simulink model "gm_IPCore_3Level_PWM"  (R2024a)
settings: Solver=VariableStepAuto  StartTime=0.0  StopTime=0.001  RelTol=1e-3
undefined symbols (not defined in the file or in its folder): f_Carrier, f_FPGA_clk, T_Carrier, T_FPGA_clk
libraries: hdlsllib x2
settings Model: PacingRate=0.100000  Creator=info  LastModifiedBy=info
settings OptimizationCC: BlockReduction=off  ConditionallyExecuteInputs=off  DefaultParameterBehavior=Inlined
settings DebuggingCC: AlgebraicLoopMsg=error  InheritedTsInSrcMsg=none  SingleTaskRateTransMsg=error
settings HardwareCC: ProdBitPerPointer=32  ProdBitPerSizeT=32  ProdBitPerPtrDiffT=32  ProdLargestAtomicFloat=None  ProdIntDivRoundTo=Undefined  ProdEndianess=Unspecified  ProdWordSize=32  ProdHWDeviceType=ASIC/FPGA->ASIC/FPGA  TargetBitPerPointer=64  TargetBitPerSizeT=64  TargetBitPerPtrDiffT=64  TargetLongLongMode=on  TargetIntDivRoundTo=Zero  TargetEndianess=LittleEndian  TargetWordSize=64  TargetHWDeviceType=Custom Processor->MATLAB Host Computer  ProdEqTarget=off

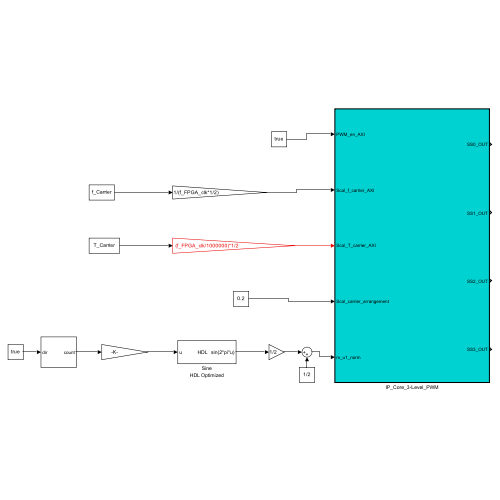
[thumbnail: Simulink's stored preview of the top-level diagram]
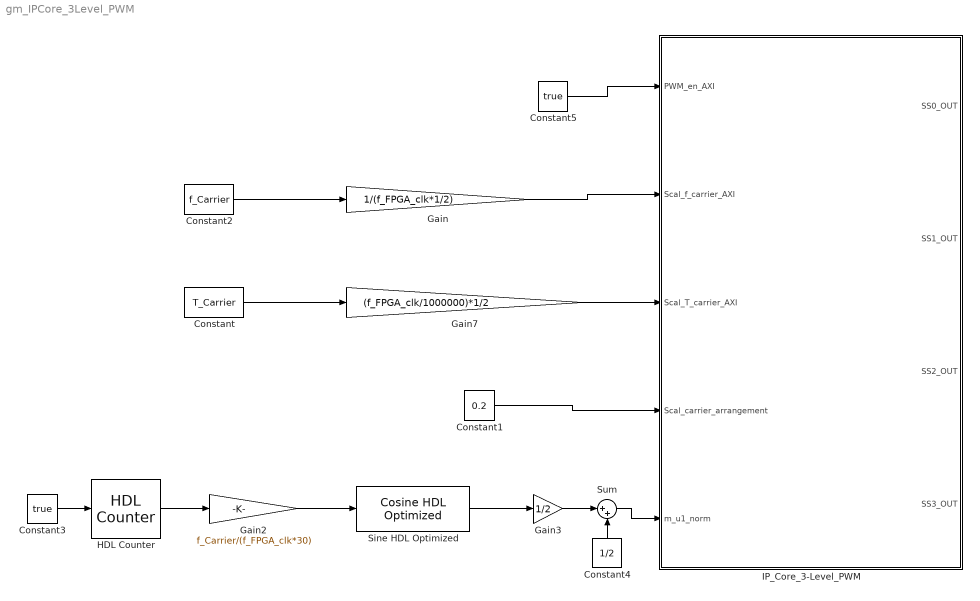
== system gm_IPCore_3Level_PWM ==
  Constant : Constant  Value=T_Carrier  SampleTime=T_FPGA_clk
  Constant1 : Constant  Value=0.2  OutDataTypeStr=double  SampleTime=T_FPGA_clk
  Constant2 : Constant  Value=f_Carrier  SampleTime=T_FPGA_clk
  Constant3 : Constant  Value=true  OutDataTypeStr=boolean  SampleTime=T_FPGA_clk
  Constant4 : Constant  Value=1/2  SampleTime=-1
  Constant5 : Constant  Value=true  SampleTime=-1
  Gain : Gain  Gain=1/(f_FPGA_clk*1/2)  OutDataTypeStr=fixdt(0,25,26)
  Gain2 : Gain  Gain=f_Carrier/(f_FPGA_clk*30)
  Gain3 : Gain  Gain=1/2
  Gain7 : Gain  Gain=(f_FPGA_clk/1000000)*1/2  OutDataTypeStr=fixdt(0,25,0)
  HDL Counter : hdlsllib/Sources/HDL Counter  CountType=Free running  CountInit=0  CountStep=1  CountMax=25  CountFromType=Initial value  CountFrom=0  CountResetPort=off  CountLoadPort=off  CountEnbPort=off  CountDirPort=on  CountHitOutputPort=off  CountDataType=Unsigned  CountWordLen=20  CountFracLen=0  CountSampTime=1
  IP_Core_3-Level_PWM : Subsystem  TreatAsAtomicUnit=on
  Sine HDL Optimized : hdlsllib/Lookup Tables/Cosine HDL Optimized  OutputFormula=sin(2*pi*u)  NumDataPoints=64  TableDataTypeStr=fixdt(0,16,15)  SimulateLUTROMDelay=off
      settings: LibrarySourceBlock=|
      | hdlsllib/Lookup
      | Tables/Sine
      | HDL Optimized
  Sum : Sum  Inputs=|++
  wires:
  Constant5/1 -> IP_Core_3-Level_PWM/1(PWM_en_AXI)
  Sum/1 -> IP_Core_3-Level_PWM/5(m_u1_norm)
  Gain3/1 -> Sum/1
  Constant4/1 -> Sum/2
  Constant3/1 -> HDL Counter/1
  HDL Counter/1 -> Gain2/1
  Gain2/1 -> Sine HDL Optimized/1
  Sine HDL Optimized/1 -> Gain3/1
  Constant1/1 -> IP_Core_3-Level_PWM/4(Scal_carrier_arrangement)
  Gain7/1 -> IP_Core_3-Level_PWM/3(Scal_T_carrier_AXI)
  Constant2/1 -> Gain/1
  Constant/1 -> Gain7/1
  Gain/1 -> IP_Core_3-Level_PWM/2(Scal_f_carrier_AXI)

== system gm_IPCore_3Level_PWM/IP_Core_3-Level_PWM ==
  note: Set pulse width in percent
  PWM_en_AXI : Inport  OutDataTypeStr=boolean  PortDimensions=1  SampleTime=1e-08
  Scal_f_carrier_AXI : Inport  Port=2  OutDataTypeStr=fixdt(0, 25, 26)  PortDimensions=1  SampleTime=1e-08
  Scal_T_carrier_AXI : Inport  Port=3  OutDataTypeStr=fixdt(0, 25, 0)  PortDimensions=1  SampleTime=1e-08
  Scal_carrier_arrangement : Inport  Port=4  OutDataTypeStr=double  PortDimensions=1  SampleTime=1e-08
  m_u1_norm : Inport  Port=5  OutDataTypeStr=double  PortDimensions=1  SampleTime=1e-08
  GenPWM : Subsystem
  Scal_f_carrier_AXI_term1 : Terminator
  SS0_OUT : Outport  SampleTime=1e-08  VectorParamsAs1DForOutWhenUnconnected=off
  SS1_OUT : Outport  Port=2  SampleTime=1e-08  VectorParamsAs1DForOutWhenUnconnected=off
  SS2_OUT : Outport  Port=3  SampleTime=1e-08  VectorParamsAs1DForOutWhenUnconnected=off
  SS3_OUT : Outport  Port=4  SampleTime=1e-08  VectorParamsAs1DForOutWhenUnconnected=off
  wires:
  PWM_en_AXI/1 -> GenPWM/1(PWM_en_AXI)
  Scal_f_carrier_AXI/1 -> Scal_f_carrier_AXI_term1/1
  Scal_T_carrier_AXI/1 -> GenPWM/2(Scal_T_carrier)
  Scal_carrier_arrangement/1 -> GenPWM/3(Scal_Carrier_arrangement)
  m_u1_norm/1 -> GenPWM/4(U1_norm)
  GenPWM/1(U1_S0) -> SS0_OUT/1
  GenPWM/2(U1_S1) -> SS1_OUT/1
  GenPWM/3(U1_S2) -> SS2_OUT/1
  GenPWM/4(U1_S3) -> SS3_OUT/1

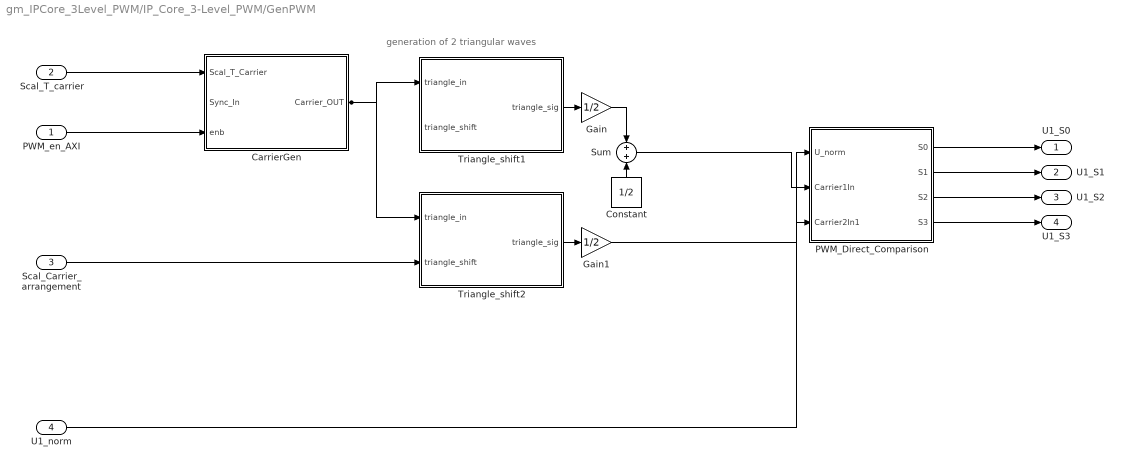
== system gm_IPCore_3Level_PWM/IP_Core_3-Level_PWM/GenPWM ==
  note: generation of 2 triangular waves
  PWM_en_AXI : Inport  OutDataTypeStr=boolean  PortDimensions=1  SampleTime=1e-08
  Scal_T_carrier : Inport  Port=2  OutDataTypeStr=fixdt(0, 25, 0)  PortDimensions=1  SampleTime=1e-08
  Scal_Carrier_arrangement : Inport  Port=3  OutDataTypeStr=double  PortDimensions=1  SampleTime=1e-08
  U1_norm : Inport  Port=4  OutDataTypeStr=double  PortDimensions=1  SampleTime=1e-08
  CarrierGen : Subsystem
  Constant : Constant  Value=1/2  OutDataTypeStr=fixdt(1,18,16)  SampleTime=T_FPGA_clk
  Gain : Gain  Gain=1/2  OutDataTypeStr=fixdt(1, 36, 33)
  Gain1 : Gain  Gain=1/2  OutDataTypeStr=fixdt(1, 36, 33)
  PWM_Direct_Comparison : Subsystem
  Sum : Sum  Inputs=+|+  OutDataTypeStr=fixdt(1, 37, 33)
  Triangle_shift1 : Subsystem
  Triangle_shift2 : Subsystem
  U1_S0 : Outport  SampleTime=1e-08
  U1_S1 : Outport  Port=2  SampleTime=1e-08
  U1_S2 : Outport  Port=3  SampleTime=1e-08
  U1_S3 : Outport  Port=4  SampleTime=1e-08
  wires:
  PWM_en_AXI/1 -> CarrierGen/3(enb)
  Scal_T_carrier/1 -> CarrierGen/1(Scal_T_Carrier)
  Scal_Carrier_arrangement/1 -> Triangle_shift2/2(triangle_shift)
  U1_norm/1 -> PWM_Direct_Comparison/1(U_norm)
  CarrierGen/1(Carrier_OUT) -> Triangle_shift1/1(triangle_in), Triangle_shift2/1(triangle_in)
  Constant/1 -> Sum/2
  Gain/1 -> Sum/1
  Gain1/1 -> PWM_Direct_Comparison/3(Carrier2In1)
  PWM_Direct_Comparison/1(S0) -> U1_S0/1
  PWM_Direct_Comparison/2(S1) -> U1_S1/1
  PWM_Direct_Comparison/3(S2) -> U1_S2/1
  PWM_Direct_Comparison/4(S3) -> U1_S3/1
  Sum/1 -> PWM_Direct_Comparison/2(Carrier1In)
  Triangle_shift1/1(triangle_sig) -> Gain/1
  Triangle_shift2/1(triangle_sig) -> Gain1/1

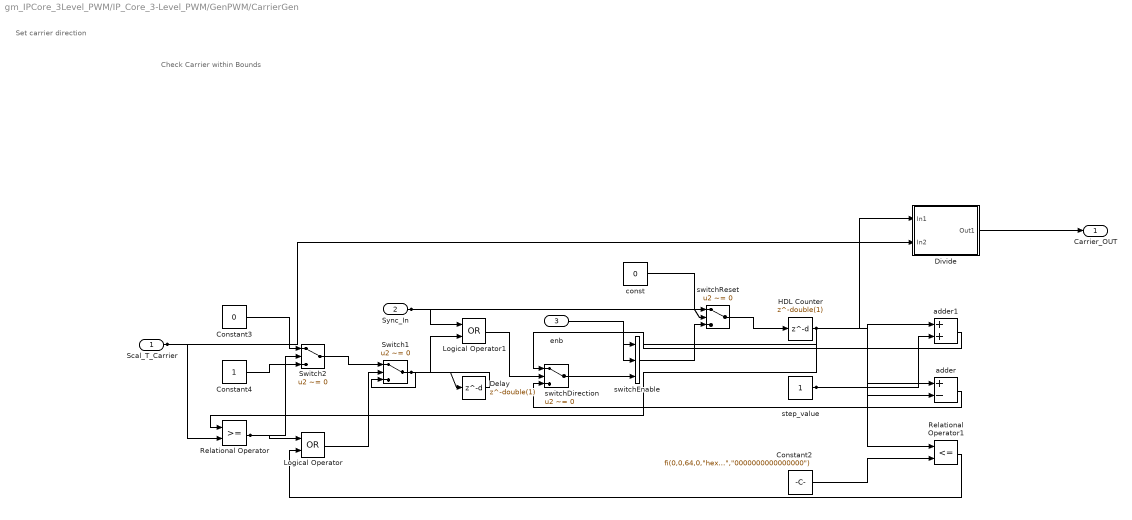
== system gm_IPCore_3Level_PWM/IP_Core_3-Level_PWM/GenPWM/CarrierGen ==
  note: Check Carrier within Bounds
  note: Set carrier direction
  Scal_T_Carrier : Inport  OutDataTypeStr=fixdt(0, 25, 0)  PortDimensions=1  SampleTime=1e-08
  Sync_In : Inport  Port=2  OutDataTypeStr=boolean  PortDimensions=1  SampleTime=1e-08
  enb : Inport  Port=3  OutDataTypeStr=boolean  PortDimensions=1  SampleTime=1e-08
  Constant2 : Constant  Value="fi(0,0,64,0,\"hex\",\"0000000000000000\")"  OutDataTypeStr=fixdt(0, 64, 0)  SampleTime=1e-08
  Constant3 : Constant  Value=0  OutDataTypeStr=boolean  SampleTime=1e-08
  Constant4 : Constant  OutDataTypeStr=boolean  SampleTime=1e-08
  Delay : Delay  DelayLength=double(1)  InitialCondition=0  SampleTime=1e-08
  Divide : Subsystem
  HDL Counter : Delay  DelayLength=double(1)  InitialCondition=0  SampleTime=1e-08
  Logical Operator : Logic  Operator=OR  AllPortsSameDT=off  OutDataTypeStr=boolean  SampleTime=1e-08
  Logical Operator1 : Logic  Operator=OR  AllPortsSameDT=off  OutDataTypeStr=boolean  SampleTime=1e-08
  Relational Operator : RelationalOperator  OutDataTypeStr=boolean  SampleTime=1e-08  InputSameDT=off
  Relational Operator1 : RelationalOperator  Operator=<=  OutDataTypeStr=boolean  SampleTime=1e-08  InputSameDT=off
  Switch1 : Switch  Criteria=u2 ~= 0  Threshold=double(0)  OutDataTypeStr=boolean  SampleTime=1e-08  SaturateOnIntegerOverflow=off  InputSameDT=off
  Switch2 : Switch  Criteria=u2 ~= 0  Threshold=double(0)  OutDataTypeStr=boolean  SampleTime=1e-08  SaturateOnIntegerOverflow=off  InputSameDT=off
  adder : Sum  Inputs=+-  OutDataTypeStr=fixdt(0, 20, 0)  AccumDataTypeStr=fixdt(0, 20, 0)  SampleTime=1e-08
  adder1 : Sum  OutDataTypeStr=fixdt(0, 20, 0)  AccumDataTypeStr=fixdt(0, 20, 0)  SampleTime=1e-08
  const : Constant  Value=0  VectorParams1D=off  OutDataTypeStr=fixdt(0, 20, 0)  SampleTime=1e-08
  step_value : Constant  VectorParams1D=off  OutDataTypeStr=fixdt(0, 20, 0)  SampleTime=1e-08
  switchDirection : Switch  Criteria=u2 ~= 0  Threshold=double(0)  OutDataTypeStr=fixdt(0, 20, 0)  SampleTime=1e-08  SaturateOnIntegerOverflow=off  InputSameDT=off
  switchEnable : MultiPortSwitch  DataPortOrder=Zero-based contiguous  Inputs=2  DiagnosticForDefault=None  zeroidx=on  OutDataTypeStr=fixdt(0, 20, 0)  SampleTime=1e-08  SaturateOnIntegerOverflow=off  InputSameDT=off
  switchReset : Switch  Criteria=u2 ~= 0  Threshold=double(0)  OutDataTypeStr=fixdt(0, 20, 0)  SampleTime=1e-08  SaturateOnIntegerOverflow=off  InputSameDT=off
  Carrier_OUT : Outport  SampleTime=1e-08
  wires:
  Scal_T_Carrier/1 -> Relational Operator/2, Divide/2(In2)
  Divide/1(Out1) -> Carrier_OUT/1
  HDL Counter/1 -> Relational Operator/1, Relational Operator1/1, adder1/1, adder/1, switchEnable/2, Divide/1(In1)
  Delay/1 -> Switch1/3
  step_value/1 -> adder1/2, adder/2
  Constant2/1 -> Relational Operator1/2
  Constant3/1 -> Switch2/1
  Constant4/1 -> Switch2/3
  Sync_In/1 -> switchReset/2, Logical Operator1/1
  enb/1 -> switchEnable/1
  const/1 -> switchReset/1
  Switch1/1 -> Delay/1, Logical Operator1/2
  switchReset/1 -> HDL Counter/1
  adder/1 -> switchDirection/3
  Relational Operator1/1 -> Logical Operator/2
  Logical Operator/1 -> Switch1/2
  Relational Operator/1 -> Switch2/2, Logical Operator/1
  Switch2/1 -> Switch1/1
  Logical Operator1/1 -> switchDirection/2
  adder1/1 -> switchDirection/1
  switchDirection/1 -> switchEnable/3
  switchEnable/1 -> switchReset/3

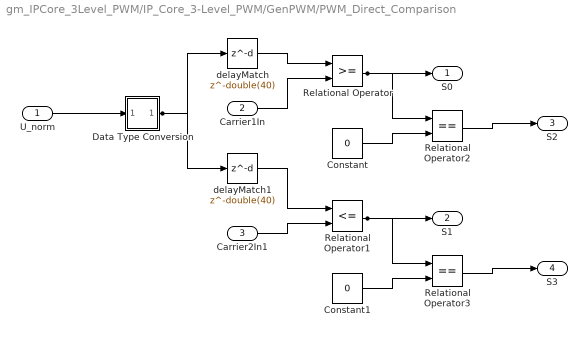
== system gm_IPCore_3Level_PWM/IP_Core_3-Level_PWM/GenPWM/PWM_Direct_Comparison ==
  U_norm : Inport  OutDataTypeStr=double  PortDimensions=1  SampleTime=1e-08
  Carrier1In : Inport  Port=2  OutDataTypeStr=fixdt(1, 37, 33)  PortDimensions=1  SampleTime=1e-08
  Carrier2In1 : Inport  Port=3  OutDataTypeStr=fixdt(1, 36, 33)  PortDimensions=1  SampleTime=1e-08
  Constant : Constant  Value=0  OutDataTypeStr=boolean  SampleTime=1e-08
  Constant1 : Constant  Value=0  OutDataTypeStr=boolean  SampleTime=1e-08
  Data Type Conversion : Subsystem
      mask Display: disp('NFP\nconv');
  Relational Operator : RelationalOperator  OutDataTypeStr=boolean  SampleTime=1e-08  InputSameDT=off
  Relational Operator1 : RelationalOperator  Operator=<=  OutDataTypeStr=boolean  SampleTime=1e-08  InputSameDT=off
  Relational Operator2 : RelationalOperator  Operator===  OutDataTypeStr=boolean  SampleTime=1e-08  InputSameDT=off
  Relational Operator3 : RelationalOperator  Operator===  OutDataTypeStr=boolean  SampleTime=1e-08  InputSameDT=off
  delayMatch : Delay  DelayLength=double(40)  InitialCondition=0  SampleTime=1e-08
  delayMatch1 : Delay  DelayLength=double(40)  InitialCondition=0  SampleTime=1e-08
  S0 : Outport  SampleTime=1e-08
  S1 : Outport  Port=2  SampleTime=1e-08
  S2 : Outport  Port=3  SampleTime=1e-08
  S3 : Outport  Port=4  SampleTime=1e-08
  wires:
  U_norm/1 -> Data Type Conversion/1(In1)
  Carrier1In/1 -> Relational Operator/2
  Carrier2In1/1 -> Relational Operator1/2
  Constant/1 -> Relational Operator2/2
  Constant1/1 -> Relational Operator3/2
  delayMatch/1 -> Relational Operator/1
  Relational Operator/1 -> Relational Operator2/1, S0/1
  Relational Operator1/1 -> Relational Operator3/1, S1/1
  Relational Operator2/1 -> S2/1
  Relational Operator3/1 -> S3/1
  Data Type Conversion/1(Out1) -> delayMatch1/1, delayMatch/1
  delayMatch1/1 -> Relational Operator1/1

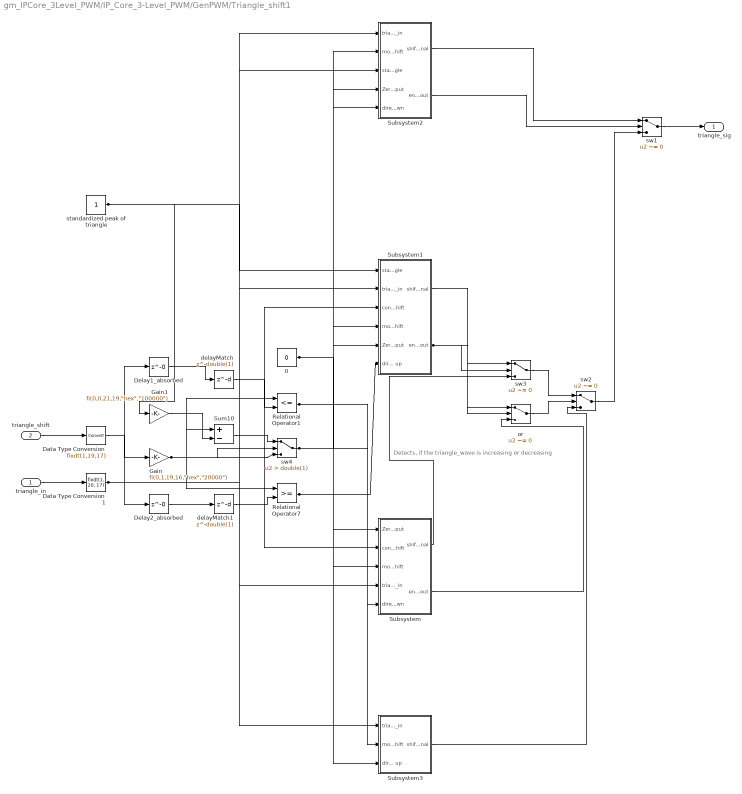
== system gm_IPCore_3Level_PWM/IP_Core_3-Level_PWM/GenPWM/Triangle_shift1 ==
  note: Detects, if the triangle_wave is increasing or decreasing
  triangle_in : Inport  OutDataTypeStr=fixdt(1, 18, 16)  PortDimensions=1  SampleTime=1e-08
  triangle_shift : Inport  Port=2  OutDataTypeStr=fixdt(1, 19, 17)  PortDimensions=1  SampleTime=1e-08
  0 : Constant  Value=0  OutDataTypeStr=boolean  SampleTime=1e-08
  Data Type Conversion : DataTypeConversion  OutDataTypeStr=fixdt(1,19,17)
  Data Type Conversion1 : DataTypeConversion  OutDataTypeStr=fixdt(1, 20, 17)  SampleTime=1e-08  SaturateOnIntegerOverflow=off  RndMeth=Floor
  Delay1_absorbed : Delay  DelayLength=0
  Delay2_absorbed : Delay  DelayLength=0
  Gain : Gain  Gain="fi(0,1,19,16,\"hex\",\"20000\")"  ParamDataTypeStr=fixdt(1, 19, 16)  OutDataTypeStr=fixdt(1, 20, 17)  SampleTime=1e-08
  Gain1 : Gain  Gain="fi(0,0,21,19,\"hex\",\"100000\")"  ParamDataTypeStr=fixdt(0, 21, 19)  OutDataTypeStr=fixdt(1, 20, 17)  SampleTime=1e-08
  Relational Operator1 : RelationalOperator  Operator=<=  OutDataTypeStr=boolean  SampleTime=1e-08  InputSameDT=off
  Relational Operator7 : RelationalOperator  OutDataTypeStr=boolean  SampleTime=1e-08  InputSameDT=off
  Subsystem : Subsystem
  Subsystem1 : Subsystem
  Subsystem2 : Subsystem
  Subsystem3 : Subsystem
  Sum10 : Sum  Inputs=+-  OutDataTypeStr=fixdt(1, 20, 17)  AccumDataTypeStr=fixdt(1, 21, 17)  SampleTime=1e-08
  delayMatch : Delay  DelayLength=double(1)  InitialCondition=0  SampleTime=1e-08
  delayMatch1 : Delay  DelayLength=double(1)  InitialCondition=0  SampleTime=1e-08
  or : Switch  Criteria=u2 ~= 0  Threshold=double(0)  OutDataTypeStr=boolean  SampleTime=1e-08  SaturateOnIntegerOverflow=off  InputSameDT=off
  standardized peak of triangle : Constant  OutDataTypeStr=fixdt(0, 21, 17)  SampleTime=1e-08
  sw1 : Switch  Criteria=u2 ~= 0  Threshold=double(0)  OutDataTypeStr=fixdt(1, 18, 16)  SampleTime=1e-08  SaturateOnIntegerOverflow=off  InputSameDT=off
  sw2 : Switch  Criteria=u2 ~= 0  Threshold=double(0)  OutDataTypeStr=fixdt(1, 21, 17)  SampleTime=1e-08  SaturateOnIntegerOverflow=off  InputSameDT=off
  sw3 : Switch  Criteria=u2 ~= 0  Threshold=double(0)  OutDataTypeStr=fixdt(1, 21, 17)  SampleTime=1e-08  SaturateOnIntegerOverflow=off  InputSameDT=off
  sw4 : Switch  Criteria=u2 > Threshold  Threshold=double(1)  OutDataTypeStr=fixdt(1, 20, 17)  SampleTime=1e-08  SaturateOnIntegerOverflow=off  InputSameDT=off
  triangle_sig : Outport  SampleTime=1e-08  VectorParamsAs1DForOutWhenUnconnected=off
  wires:
  triangle_in/1 -> Data Type Conversion1/1
  triangle_shift/1 -> Data Type Conversion/1
  0/1 -> Subsystem2/4(Zero_input), Subsystem1/5(Zero_input), Subsystem/1(Zero_input)
  Data Type Conversion/1 -> Gain/1
  Data Type Conversion1/1 -> Relational Operator7/1, Relational Operator1/1, Subsystem3/1(triangle_in), Subsystem2/1(triangle_in), Subsystem/4(triangle_in), Subsystem1/2(triangle_in), Delay1_absorbed/1, Delay2_absorbed/1
  delayMatch/1 -> Relational Operator1/2
  delayMatch1/1 -> Relational Operator7/2
  Gain/1 -> sw4/3, sw4/2, Sum10/1, Subsystem/2(converted triangle_shift), Subsystem1/3(converted triangle_shift)
  Gain1/1 -> Sum10/2
  Relational Operator1/1 -> Subsystem/5(direction down), Subsystem2/5(direction down)
  Relational Operator7/1 -> Subsystem1/6(direction up), Subsystem3/3(direction up)
  Subsystem/1(shifted triangle_in signal) -> sw3/3
  Subsystem/2(enable_out) -> or/3
  Subsystem1/1(shifted triangle_in signal) -> sw3/1
  Subsystem1/2(enable_out) -> sw3/2, or/2, or/1
  Subsystem2/1(shifted triangle_in signal) -> sw1/1
  Subsystem2/2(enable_out) -> sw1/2
  Subsystem3/1(shifted triangle_in signal) -> sw2/3
  Sum10/1 -> sw4/1
  or/1 -> sw2/2
  standardized peak of triangle/1 -> Gain1/1, Subsystem2/3(standardized peak of triangle), Subsystem1/1(standardized peak of triangle)
  sw1/1 -> triangle_sig/1
  sw2/1 -> sw1/3
  sw3/1 -> sw2/1
  sw4/1 -> Subsystem3/2(modified triangle_shift), Subsystem/3(modified triangle_shift), Subsystem1/4(modified triangle_shift), Subsystem2/2(modified triangle_shift)
  Delay1_absorbed/1 -> delayMatch/1
  Delay2_absorbed/1 -> delayMatch1/1

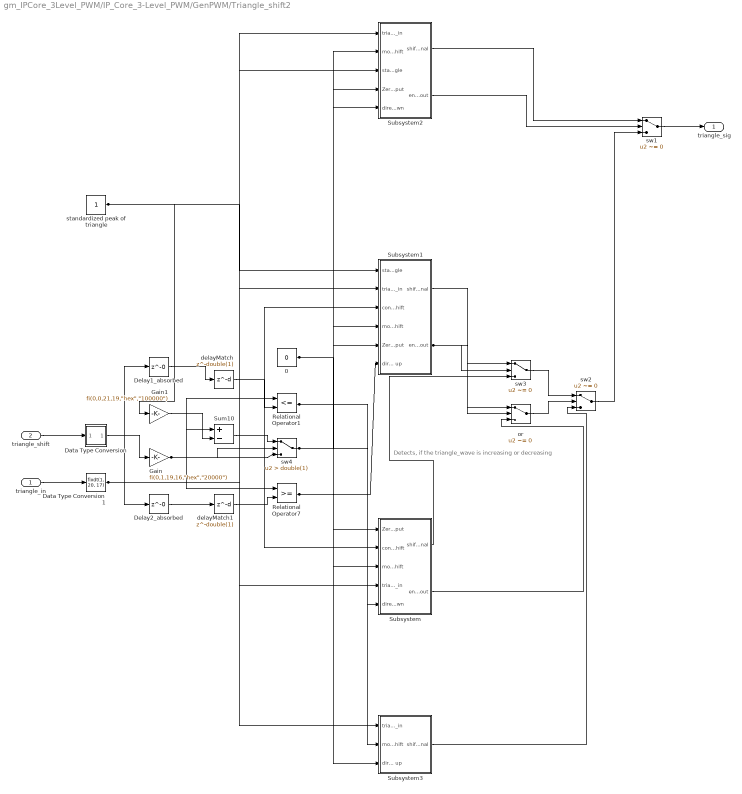
== system gm_IPCore_3Level_PWM/IP_Core_3-Level_PWM/GenPWM/Triangle_shift2 ==
  note: Detects, if the triangle_wave is increasing or decreasing
  triangle_in : Inport  OutDataTypeStr=fixdt(1, 18, 16)  PortDimensions=1  SampleTime=1e-08
  triangle_shift : Inport  Port=2  OutDataTypeStr=double  PortDimensions=1  SampleTime=1e-08
  0 : Constant  Value=0  OutDataTypeStr=boolean  SampleTime=1e-08
  Data Type Conversion : Subsystem
      mask Display: disp('NFP\nconv');
  Data Type Conversion1 : DataTypeConversion  OutDataTypeStr=fixdt(1, 20, 17)  SampleTime=1e-08  SaturateOnIntegerOverflow=off  RndMeth=Floor
  Delay1_absorbed : Delay  DelayLength=0
  Delay2_absorbed : Delay  DelayLength=0
  Gain : Gain  Gain="fi(0,1,19,16,\"hex\",\"20000\")"  ParamDataTypeStr=fixdt(1, 19, 16)  OutDataTypeStr=fixdt(1, 20, 17)  SampleTime=1e-08
  Gain1 : Gain  Gain="fi(0,0,21,19,\"hex\",\"100000\")"  ParamDataTypeStr=fixdt(0, 21, 19)  OutDataTypeStr=fixdt(1, 20, 17)  SampleTime=1e-08
  Relational Operator1 : RelationalOperator  Operator=<=  OutDataTypeStr=boolean  SampleTime=1e-08  InputSameDT=off
  Relational Operator7 : RelationalOperator  OutDataTypeStr=boolean  SampleTime=1e-08  InputSameDT=off
  Subsystem : Subsystem
  Subsystem1 : Subsystem
  Subsystem2 : Subsystem
  Subsystem3 : Subsystem
  Sum10 : Sum  Inputs=+-  OutDataTypeStr=fixdt(1, 20, 17)  AccumDataTypeStr=fixdt(1, 21, 17)  SampleTime=1e-08
  delayMatch : Delay  DelayLength=double(1)  InitialCondition=0  SampleTime=1e-08
  delayMatch1 : Delay  DelayLength=double(1)  InitialCondition=0  SampleTime=1e-08
  or : Switch  Criteria=u2 ~= 0  Threshold=double(0)  OutDataTypeStr=boolean  SampleTime=1e-08  SaturateOnIntegerOverflow=off  InputSameDT=off
  standardized peak of triangle : Constant  OutDataTypeStr=fixdt(0, 21, 17)  SampleTime=1e-08
  sw1 : Switch  Criteria=u2 ~= 0  Threshold=double(0)  OutDataTypeStr=fixdt(1, 18, 16)  SampleTime=1e-08  SaturateOnIntegerOverflow=off  InputSameDT=off
  sw2 : Switch  Criteria=u2 ~= 0  Threshold=double(0)  OutDataTypeStr=fixdt(1, 21, 17)  SampleTime=1e-08  SaturateOnIntegerOverflow=off  InputSameDT=off
  sw3 : Switch  Criteria=u2 ~= 0  Threshold=double(0)  OutDataTypeStr=fixdt(1, 21, 17)  SampleTime=1e-08  SaturateOnIntegerOverflow=off  InputSameDT=off
  sw4 : Switch  Criteria=u2 > Threshold  Threshold=double(1)  OutDataTypeStr=fixdt(1, 20, 17)  SampleTime=1e-08  SaturateOnIntegerOverflow=off  InputSameDT=off
  triangle_sig : Outport  SampleTime=1e-08  VectorParamsAs1DForOutWhenUnconnected=off
  wires:
  triangle_in/1 -> Data Type Conversion1/1
  triangle_shift/1 -> Data Type Conversion/1(In1)
  0/1 -> Subsystem2/4(Zero_input), Subsystem1/5(Zero_input), Subsystem/1(Zero_input)
  Data Type Conversion1/1 -> Relational Operator7/1, Relational Operator1/1, Subsystem3/1(triangle_in), Subsystem2/1(triangle_in), Subsystem/4(triangle_in), Subsystem1/2(triangle_in), Delay2_absorbed/1, Delay1_absorbed/1
  delayMatch/1 -> Relational Operator1/2
  delayMatch1/1 -> Relational Operator7/2
  Gain/1 -> sw4/3, sw4/2, Sum10/1, Subsystem/2(converted triangle_shift), Subsystem1/3(converted triangle_shift)
  Gain1/1 -> Sum10/2
  Relational Operator1/1 -> Subsystem/5(direction down), Subsystem2/5(direction down)
  Relational Operator7/1 -> Subsystem1/6(direction up), Subsystem3/3(direction up)
  Subsystem/1(shifted triangle_in signal) -> sw3/3
  Subsystem/2(enable_out) -> or/3
  Subsystem1/1(shifted triangle_in signal) -> sw3/1
  Subsystem1/2(enable_out) -> sw3/2, or/2, or/1
  Subsystem2/1(shifted triangle_in signal) -> sw1/1
  Subsystem2/2(enable_out) -> sw1/2
  Subsystem3/1(shifted triangle_in signal) -> sw2/3
  Sum10/1 -> sw4/1
  or/1 -> sw2/2
  standardized peak of triangle/1 -> Gain1/1, Subsystem2/3(standardized peak of triangle), Subsystem1/1(standardized peak of triangle)
  sw1/1 -> triangle_sig/1
  sw2/1 -> sw1/3
  sw3/1 -> sw2/1
  sw4/1 -> Subsystem3/2(modified triangle_shift), Subsystem/3(modified triangle_shift), Subsystem1/4(modified triangle_shift), Subsystem2/2(modified triangle_shift)
  Data Type Conversion/1(Out1) -> Gain/1
  Delay1_absorbed/1 -> delayMatch/1
  Delay2_absorbed/1 -> delayMatch1/1

== system gm_IPCore_3Level_PWM/IP_Core_3-Level_PWM/GenPWM/CarrierGen/Divide ==
  In1 : Inport
  In2 : Inport  Port=2
  Divide : Product  Inputs=*/  OutDataTypeStr=fixdt(1,18,16)  RndMeth=Zero  SaturateOnIntegerOverflow=on
  Divide_pd1 : Delay  DelayLength=46
  Out1 : Outport
  wires:
  In2/1 -> Divide/2
  In1/1 -> Divide/1
  Divide_pd1/1 -> Out1/1
  Divide/1 -> Divide_pd1/1

== system gm_IPCore_3Level_PWM/IP_Core_3-Level_PWM/GenPWM/PWM_Direct_Comparison/Data Type Conversion ==
  In1 : Inport
  Data Type Conversion : DataTypeConversion  OutDataTypeStr=fixdt(1, 20, 17)  RndMeth=Nearest  SampleTime=1e-08  SaturateOnIntegerOverflow=off
  Data Type Conversion_pd1 : Delay  DelayLength=6
  Out1 : Outport
  wires:
  In1/1 -> Data Type Conversion/1
  Data Type Conversion/1 -> Data Type Conversion_pd1/1
  Data Type Conversion_pd1/1 -> Out1/1

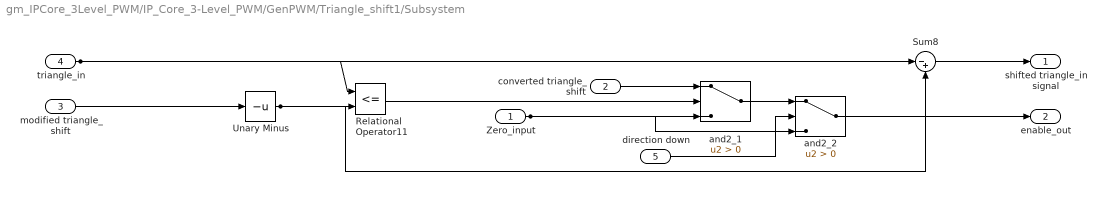
== system gm_IPCore_3Level_PWM/IP_Core_3-Level_PWM/GenPWM/Triangle_shift1/Subsystem ==
  Zero_input : Inport  OutDataTypeStr=boolean  PortDimensions=1  SampleTime=1e-08
  converted triangle_shift : Inport  Port=2  OutDataTypeStr=fixdt(1, 20, 17)  PortDimensions=1  SampleTime=1e-08
  modified triangle_shift : Inport  Port=3  OutDataTypeStr=fixdt(1, 20, 17)  PortDimensions=1  SampleTime=1e-08
  triangle_in : Inport  Port=4  OutDataTypeStr=fixdt(1, 20, 17)  PortDimensions=1  SampleTime=1e-08
  direction down : Inport  Port=5  OutDataTypeStr=boolean  PortDimensions=1  SampleTime=1e-08
  Relational Operator11 : RelationalOperator  Operator=<=  OutDataTypeStr=boolean  InputSameDT=off
  Sum8 : Sum  Inputs=|-+  OutDataTypeStr=fixdt(1, 21, 17)
  Unary Minus : UnaryMinus
  and2_1 : Switch  Criteria=u2 > Threshold  OutDataTypeStr=boolean  SaturateOnIntegerOverflow=off  InputSameDT=off
  and2_2 : Switch  Criteria=u2 > Threshold  OutDataTypeStr=boolean  SaturateOnIntegerOverflow=off  InputSameDT=off
  shifted triangle_in signal : Outport  SampleTime=1e-08
  enable_out : Outport  Port=2  SampleTime=1e-08
  wires:
  Zero_input/1 -> and2_2/3, and2_1/3
  converted triangle_shift/1 -> and2_1/1
  modified triangle_shift/1 -> Unary Minus/1
  triangle_in/1 -> Sum8/1, Relational Operator11/1
  direction down/1 -> and2_2/2
  Relational Operator11/1 -> and2_1/2
  Sum8/1 -> shifted triangle_in signal/1
  Unary Minus/1 -> Sum8/2, Relational Operator11/2
  and2_1/1 -> and2_2/1
  and2_2/1 -> enable_out/1

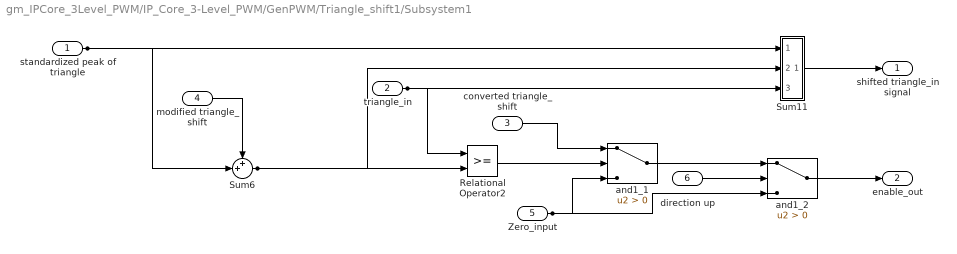
== system gm_IPCore_3Level_PWM/IP_Core_3-Level_PWM/GenPWM/Triangle_shift1/Subsystem1 ==
  standardized peak of triangle : Inport  OutDataTypeStr=fixdt(0, 21, 17)  PortDimensions=1  SampleTime=1e-08
  triangle_in : Inport  Port=2  OutDataTypeStr=fixdt(1, 20, 17)  PortDimensions=1  SampleTime=1e-08
  converted triangle_shift : Inport  Port=3  OutDataTypeStr=fixdt(1, 20, 17)  PortDimensions=1  SampleTime=1e-08
  modified triangle_shift : Inport  Port=4  OutDataTypeStr=fixdt(1, 20, 17)  PortDimensions=1  SampleTime=1e-08
  Zero_input : Inport  Port=5  OutDataTypeStr=boolean  PortDimensions=1  SampleTime=1e-08
  direction up : Inport  Port=6  OutDataTypeStr=boolean  PortDimensions=1  SampleTime=1e-08
  Relational Operator2 : RelationalOperator  OutDataTypeStr=boolean  InputSameDT=off
  Sum11 : Subsystem
  Sum6 : Sum  Inputs=++|  OutDataTypeStr=fixdt(1, 23, 17)
  and1_1 : Switch  Criteria=u2 > Threshold  OutDataTypeStr=boolean  SaturateOnIntegerOverflow=off  InputSameDT=off
  and1_2 : Switch  Criteria=u2 > Threshold  OutDataTypeStr=boolean  SaturateOnIntegerOverflow=off  InputSameDT=off
  shifted triangle_in signal : Outport  SampleTime=1e-08
  enable_out : Outport  Port=2  SampleTime=1e-08
  wires:
  standardized peak of triangle/1 -> Sum6/2, Sum11/1(In1)
  triangle_in/1 -> Sum11/3(In3), Relational Operator2/1
  converted triangle_shift/1 -> and1_1/1
  modified triangle_shift/1 -> Sum6/1
  Zero_input/1 -> and1_2/3, and1_1/3
  direction up/1 -> and1_2/2
  Relational Operator2/1 -> and1_1/2
  Sum11/1(Out1) -> shifted triangle_in signal/1
  Sum6/1 -> Sum11/2(In2), Relational Operator2/2
  and1_1/1 -> and1_2/1
  and1_2/1 -> enable_out/1

== system gm_IPCore_3Level_PWM/IP_Core_3-Level_PWM/GenPWM/Triangle_shift1/Subsystem2 ==
  triangle_in : Inport  OutDataTypeStr=fixdt(1, 20, 17)  PortDimensions=1  SampleTime=1e-08
  modified triangle_shift : Inport  Port=2  OutDataTypeStr=fixdt(1, 20, 17)  PortDimensions=1  SampleTime=1e-08
  standardized peak of triangle : Inport  Port=3  OutDataTypeStr=fixdt(0, 21, 17)  PortDimensions=1  SampleTime=1e-08
  Zero_input : Inport  Port=4  OutDataTypeStr=boolean  PortDimensions=1  SampleTime=1e-08
  direction down : Inport  Port=5  OutDataTypeStr=boolean  PortDimensions=1  SampleTime=1e-08
  Relational Operator9 : RelationalOperator  OutDataTypeStr=boolean  InputSameDT=off
  Sum1 : Sum  Inputs=|-+  OutDataTypeStr=fixdt(1, 23, 17)
  Sum5 : Subsystem
  and : Switch  Criteria=u2 > Threshold  OutDataTypeStr=boolean  SaturateOnIntegerOverflow=off  InputSameDT=off
  shifted triangle_in signal : Outport  SampleTime=1e-08
  enable_out : Outport  Port=2  SampleTime=1e-08
  wires:
  triangle_in/1 -> Sum5/3(In3), Relational Operator9/1
  modified triangle_shift/1 -> Sum1/1
  standardized peak of triangle/1 -> Sum5/2(In2), Sum1/2
  Zero_input/1 -> and/3
  direction down/1 -> and/2
  Relational Operator9/1 -> and/1
  Sum1/1 -> Sum5/1(In1), Relational Operator9/2
  Sum5/1(Out1) -> shifted triangle_in signal/1
  and/1 -> enable_out/1

== system gm_IPCore_3Level_PWM/IP_Core_3-Level_PWM/GenPWM/Triangle_shift1/Subsystem3 ==
  triangle_in : Inport  OutDataTypeStr=fixdt(1, 20, 17)  PortDimensions=1  SampleTime=1e-08
  modified triangle_shift : Inport  Port=2  OutDataTypeStr=fixdt(1, 20, 17)  PortDimensions=1  SampleTime=1e-08
  direction up : Inport  Port=3  OutDataTypeStr=boolean  PortDimensions=1  SampleTime=1e-08
  Relational Operator6 : RelationalOperator  Operator=<=  OutDataTypeStr=boolean  InputSameDT=off
  Sum2 : Sum  Inputs=|-+  OutDataTypeStr=fixdt(1, 21, 17)
  Sum3 : Sum  Inputs=|+-  OutDataTypeStr=fixdt(1, 21, 17)
  Sum4 : Sum  Inputs=|++  OutDataTypeStr=fixdt(1, 21, 17)
  Switch3 : Switch  Criteria=u2 > Threshold  OutDataTypeStr=fixdt(1, 21, 17)  SaturateOnIntegerOverflow=off  InputSameDT=off
  sw : Switch  Criteria=u2 > Threshold  OutDataTypeStr=fixdt(1, 21, 17)  SaturateOnIntegerOverflow=off  InputSameDT=off
  shifted triangle_in signal : Outport  SampleTime=1e-08
  wires:
  triangle_in/1 -> Sum4/2, Sum3/1, Sum2/1, Relational Operator6/1
  modified triangle_shift/1 -> Sum4/1, Sum3/2, Sum2/2, Relational Operator6/2
  direction up/1 -> sw/2
  Relational Operator6/1 -> Switch3/2
  Sum2/1 -> Switch3/1
  Sum3/1 -> Switch3/3
  Sum4/1 -> sw/3
  Switch3/1 -> sw/1
  sw/1 -> shifted triangle_in signal/1

== system gm_IPCore_3Level_PWM/IP_Core_3-Level_PWM/GenPWM/Triangle_shift2/Data Type Conversion ==
  In1 : Inport
  Data Type Conversion : DataTypeConversion  OutDataTypeStr=fixdt(1, 19, 17)  SampleTime=1e-08  SaturateOnIntegerOverflow=off  RndMeth=Floor
  Data Type Conversion_pd1 : Delay  DelayLength=6
  Out1 : Outport
  wires:
  In1/1 -> Data Type Conversion/1
  Data Type Conversion/1 -> Data Type Conversion_pd1/1
  Data Type Conversion_pd1/1 -> Out1/1

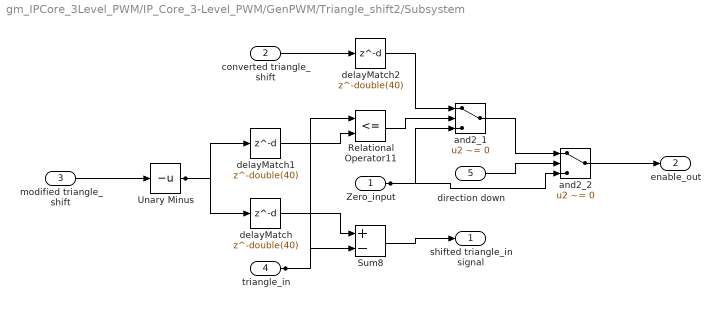
== system gm_IPCore_3Level_PWM/IP_Core_3-Level_PWM/GenPWM/Triangle_shift2/Subsystem ==
  Zero_input : Inport  OutDataTypeStr=boolean  PortDimensions=1  SampleTime=1e-08
  converted triangle_shift : Inport  Port=2  OutDataTypeStr=fixdt(1, 20, 17)  PortDimensions=1  SampleTime=1e-08
  modified triangle_shift : Inport  Port=3  OutDataTypeStr=fixdt(1, 20, 17)  PortDimensions=1  SampleTime=1e-08
  triangle_in : Inport  Port=4  OutDataTypeStr=fixdt(1, 20, 17)  PortDimensions=1  SampleTime=1e-08
  direction down : Inport  Port=5  OutDataTypeStr=boolean  PortDimensions=1  SampleTime=1e-08
  Relational Operator11 : RelationalOperator  Operator=<=  OutDataTypeStr=boolean  SampleTime=1e-08  InputSameDT=off
  Sum8 : Sum  Inputs=+-  OutDataTypeStr=fixdt(1, 21, 17)  AccumDataTypeStr=fixdt(1, 21, 17)  SampleTime=1e-08
  Unary Minus : UnaryMinus  SampleTime=1e-08
  and2_1 : Switch  Criteria=u2 ~= 0  Threshold=double(0)  OutDataTypeStr=boolean  SampleTime=1e-08  SaturateOnIntegerOverflow=off  InputSameDT=off
  and2_2 : Switch  Criteria=u2 ~= 0  Threshold=double(0)  OutDataTypeStr=boolean  SampleTime=1e-08  SaturateOnIntegerOverflow=off  InputSameDT=off
  delayMatch : Delay  DelayLength=double(40)  InitialCondition=0  SampleTime=1e-08
  delayMatch1 : Delay  DelayLength=double(40)  InitialCondition=0  SampleTime=1e-08
  delayMatch2 : Delay  DelayLength=double(40)  InitialCondition=0  SampleTime=1e-08
  shifted triangle_in signal : Outport  SampleTime=1e-08
  enable_out : Outport  Port=2  SampleTime=1e-08
  wires:
  Zero_input/1 -> and2_2/3, and2_1/3
  delayMatch2/1 -> and2_1/1
  modified triangle_shift/1 -> Unary Minus/1
  triangle_in/1 -> Sum8/2, Relational Operator11/1
  direction down/1 -> and2_2/2
  Relational Operator11/1 -> and2_1/2
  Sum8/1 -> shifted triangle_in signal/1
  delayMatch/1 -> Sum8/1
  and2_1/1 -> and2_2/1
  and2_2/1 -> enable_out/1
  delayMatch1/1 -> Relational Operator11/2
  Unary Minus/1 -> delayMatch1/1, delayMatch/1
  converted triangle_shift/1 -> delayMatch2/1

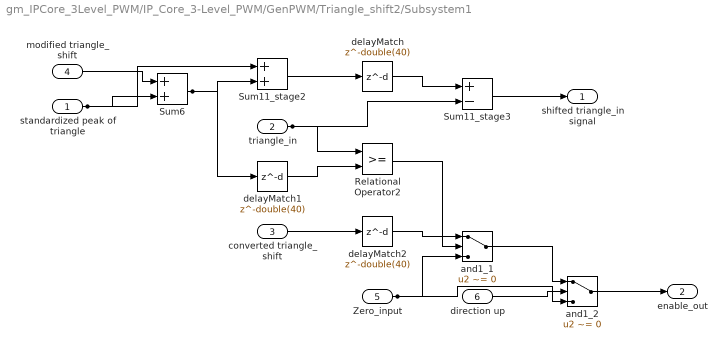
== system gm_IPCore_3Level_PWM/IP_Core_3-Level_PWM/GenPWM/Triangle_shift2/Subsystem1 ==
  standardized peak of triangle : Inport  OutDataTypeStr=fixdt(0, 21, 17)  PortDimensions=1  SampleTime=1e-08
  triangle_in : Inport  Port=2  OutDataTypeStr=fixdt(1, 20, 17)  PortDimensions=1  SampleTime=1e-08
  converted triangle_shift : Inport  Port=3  OutDataTypeStr=fixdt(1, 20, 17)  PortDimensions=1  SampleTime=1e-08
  modified triangle_shift : Inport  Port=4  OutDataTypeStr=fixdt(1, 20, 17)  PortDimensions=1  SampleTime=1e-08
  Zero_input : Inport  Port=5  OutDataTypeStr=boolean  PortDimensions=1  SampleTime=1e-08
  direction up : Inport  Port=6  OutDataTypeStr=boolean  PortDimensions=1  SampleTime=1e-08
  Relational Operator2 : RelationalOperator  OutDataTypeStr=boolean  SampleTime=1e-08  InputSameDT=off
  Sum11_stage2 : Sum  OutDataTypeStr=fixdt(1, 24, 17)  AccumDataTypeStr=fixdt(1, 24, 17)  SampleTime=1e-08
  Sum11_stage3 : Sum  Inputs=+-  OutDataTypeStr=fixdt(1, 21, 17)  AccumDataTypeStr=fixdt(1, 24, 17)  SampleTime=1e-08
  Sum6 : Sum  OutDataTypeStr=fixdt(1, 23, 17)  AccumDataTypeStr=fixdt(1, 23, 17)  SampleTime=1e-08
  and1_1 : Switch  Criteria=u2 ~= 0  Threshold=double(0)  OutDataTypeStr=boolean  SampleTime=1e-08  SaturateOnIntegerOverflow=off  InputSameDT=off
  and1_2 : Switch  Criteria=u2 ~= 0  Threshold=double(0)  OutDataTypeStr=boolean  SampleTime=1e-08  SaturateOnIntegerOverflow=off  InputSameDT=off
  delayMatch : Delay  DelayLength=double(40)  InitialCondition=0  SampleTime=1e-08
  delayMatch1 : Delay  DelayLength=double(40)  InitialCondition=0  SampleTime=1e-08
  delayMatch2 : Delay  DelayLength=double(40)  InitialCondition=0  SampleTime=1e-08
  shifted triangle_in signal : Outport  SampleTime=1e-08
  enable_out : Outport  Port=2  SampleTime=1e-08
  wires:
  standardized peak of triangle/1 -> Sum6/2, Sum11_stage2/1
  triangle_in/1 -> Sum11_stage3/2, Relational Operator2/1
  delayMatch2/1 -> and1_1/1
  modified triangle_shift/1 -> Sum6/1
  Zero_input/1 -> and1_2/3, and1_1/3
  direction up/1 -> and1_2/2
  Relational Operator2/1 -> and1_1/2
  Sum11_stage3/1 -> shifted triangle_in signal/1
  delayMatch1/1 -> Relational Operator2/2
  and1_1/1 -> and1_2/1
  and1_2/1 -> enable_out/1
  delayMatch/1 -> Sum11_stage3/1
  Sum11_stage2/1 -> delayMatch/1
  Sum6/1 -> delayMatch1/1, Sum11_stage2/2
  converted triangle_shift/1 -> delayMatch2/1

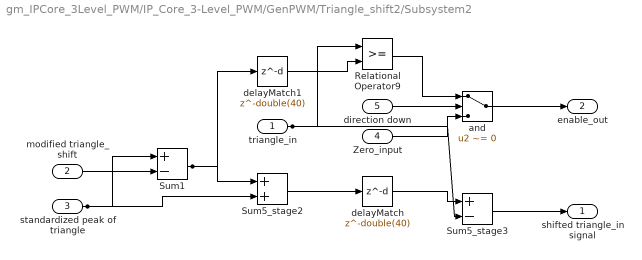
== system gm_IPCore_3Level_PWM/IP_Core_3-Level_PWM/GenPWM/Triangle_shift2/Subsystem2 ==
  triangle_in : Inport  OutDataTypeStr=fixdt(1, 20, 17)  PortDimensions=1  SampleTime=1e-08
  modified triangle_shift : Inport  Port=2  OutDataTypeStr=fixdt(1, 20, 17)  PortDimensions=1  SampleTime=1e-08
  standardized peak of triangle : Inport  Port=3  OutDataTypeStr=fixdt(0, 21, 17)  PortDimensions=1  SampleTime=1e-08
  Zero_input : Inport  Port=4  OutDataTypeStr=boolean  PortDimensions=1  SampleTime=1e-08
  direction down : Inport  Port=5  OutDataTypeStr=boolean  PortDimensions=1  SampleTime=1e-08
  Relational Operator9 : RelationalOperator  OutDataTypeStr=boolean  SampleTime=1e-08  InputSameDT=off
  Sum1 : Sum  Inputs=+-  OutDataTypeStr=fixdt(1, 23, 17)  AccumDataTypeStr=fixdt(1, 23, 17)  SampleTime=1e-08
  Sum5_stage2 : Sum  OutDataTypeStr=fixdt(1, 24, 17)  AccumDataTypeStr=fixdt(1, 24, 17)  SampleTime=1e-08
  Sum5_stage3 : Sum  Inputs=+-  OutDataTypeStr=fixdt(1, 21, 17)  AccumDataTypeStr=fixdt(1, 24, 17)  SampleTime=1e-08
  and : Switch  Criteria=u2 ~= 0  Threshold=double(0)  OutDataTypeStr=boolean  SampleTime=1e-08  SaturateOnIntegerOverflow=off  InputSameDT=off
  delayMatch : Delay  DelayLength=double(40)  InitialCondition=0  SampleTime=1e-08
  delayMatch1 : Delay  DelayLength=double(40)  InitialCondition=0  SampleTime=1e-08
  shifted triangle_in signal : Outport  SampleTime=1e-08
  enable_out : Outport  Port=2  SampleTime=1e-08
  wires:
  triangle_in/1 -> Sum5_stage3/2, Relational Operator9/1
  modified triangle_shift/1 -> Sum1/2
  standardized peak of triangle/1 -> Sum5_stage2/2, Sum1/1
  Zero_input/1 -> and/3
  direction down/1 -> and/2
  Relational Operator9/1 -> and/1
  delayMatch1/1 -> Relational Operator9/2
  Sum5_stage3/1 -> shifted triangle_in signal/1
  and/1 -> enable_out/1
  delayMatch/1 -> Sum5_stage3/1
  Sum5_stage2/1 -> delayMatch/1
  Sum1/1 -> delayMatch1/1, Sum5_stage2/1

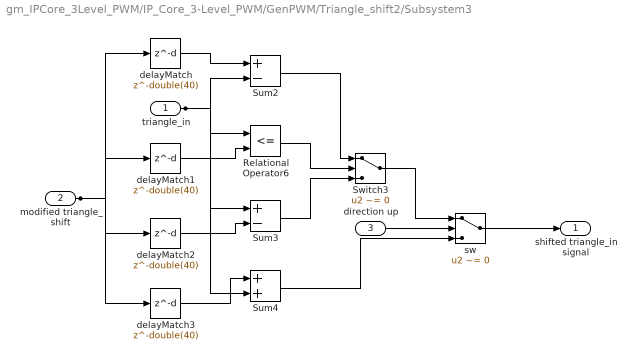
== system gm_IPCore_3Level_PWM/IP_Core_3-Level_PWM/GenPWM/Triangle_shift2/Subsystem3 ==
  triangle_in : Inport  OutDataTypeStr=fixdt(1, 20, 17)  PortDimensions=1  SampleTime=1e-08
  modified triangle_shift : Inport  Port=2  OutDataTypeStr=fixdt(1, 20, 17)  PortDimensions=1  SampleTime=1e-08
  direction up : Inport  Port=3  OutDataTypeStr=boolean  PortDimensions=1  SampleTime=1e-08
  Relational Operator6 : RelationalOperator  Operator=<=  OutDataTypeStr=boolean  SampleTime=1e-08  InputSameDT=off
  Sum2 : Sum  Inputs=+-  OutDataTypeStr=fixdt(1, 21, 17)  AccumDataTypeStr=fixdt(1, 21, 17)  SampleTime=1e-08
  Sum3 : Sum  Inputs=+-  OutDataTypeStr=fixdt(1, 21, 17)  AccumDataTypeStr=fixdt(1, 21, 17)  SampleTime=1e-08
  Sum4 : Sum  OutDataTypeStr=fixdt(1, 21, 17)  AccumDataTypeStr=fixdt(1, 21, 17)  SampleTime=1e-08
  Switch3 : Switch  Criteria=u2 ~= 0  Threshold=double(0)  OutDataTypeStr=fixdt(1, 21, 17)  SampleTime=1e-08  SaturateOnIntegerOverflow=off  InputSameDT=off
  delayMatch{,1..3} (4 alike) : Delay  DelayLength=double(40)  InitialCondition=0  SampleTime=1e-08
  sw : Switch  Criteria=u2 ~= 0  Threshold=double(0)  OutDataTypeStr=fixdt(1, 21, 17)  SampleTime=1e-08  SaturateOnIntegerOverflow=off  InputSameDT=off
  shifted triangle_in signal : Outport  SampleTime=1e-08
  wires:
  triangle_in/1 -> Sum4/2, Sum3/1, Sum2/2, Relational Operator6/1
  delayMatch/1 -> Sum2/1
  direction up/1 -> sw/2
  Relational Operator6/1 -> Switch3/2
  Sum2/1 -> Switch3/1
  Sum3/1 -> Switch3/3
  Sum4/1 -> sw/3
  Switch3/1 -> sw/1
  sw/1 -> shifted triangle_in signal/1
  delayMatch1/1 -> Relational Operator6/2
  delayMatch2/1 -> Sum3/2
  delayMatch3/1 -> Sum4/1
  modified triangle_shift/1 -> delayMatch3/1, delayMatch2/1, delayMatch1/1, delayMatch/1

== system gm_IPCore_3Level_PWM/IP_Core_3-Level_PWM/GenPWM/Triangle_shift1/Subsystem1/Sum11 ==
  In1 : Inport  OutDataTypeStr=fixdt(0,21,17)
  In2 : Inport  Port=2  OutDataTypeStr=fixdt(1,23,17)
  In3 : Inport  Port=3  OutDataTypeStr=fixdt(1,20,17)
  Sum2 : Sum  OutDataTypeStr=fixdt(1,24,17)  AccumDataTypeStr=fixdt(1,24,17)
  Sum3 : Sum  Inputs=+-  OutDataTypeStr=fixdt(1,21,17)  AccumDataTypeStr=fixdt(1,24,17)
  Out1 : Outport
  wires:
  In1/1 -> Sum2/1
  In2/1 -> Sum2/2
  Sum2/1 -> Sum3/1
  In3/1 -> Sum3/2
  Sum3/1 -> Out1/1

== system gm_IPCore_3Level_PWM/IP_Core_3-Level_PWM/GenPWM/Triangle_shift1/Subsystem2/Sum5 ==
  In1 : Inport  OutDataTypeStr=fixdt(1,23,17)
  In2 : Inport  Port=2  OutDataTypeStr=fixdt(0,21,17)
  In3 : Inport  Port=3  OutDataTypeStr=fixdt(1,20,17)
  Sum2 : Sum  OutDataTypeStr=fixdt(1,24,17)  AccumDataTypeStr=fixdt(1,24,17)
  Sum3 : Sum  Inputs=+-  OutDataTypeStr=fixdt(1,21,17)  AccumDataTypeStr=fixdt(1,24,17)
  Out1 : Outport
  wires:
  In1/1 -> Sum2/1
  In2/1 -> Sum2/2
  Sum2/1 -> Sum3/1
  In3/1 -> Sum3/2
  Sum3/1 -> Out1/1
